simulink model "project"  (R2022b)
settings: Solver=FixedStepDiscrete  StartTime=0.0  StopTime=inf  RelTol=1e-3
undefined symbols (not defined in the file): dfilt, fdesignblkfcn, gcbh
libraries: audiofilters x12, dspsnks4 x6, dsparch4 x6, dspvision x6, dspfdesign x3, simulink x3
settings Model: Creator=KT  LastModifiedBy=KT
settings SolverCC: AlgebraicLoopSolver=TrustRegion  AutoInsertRateTranBlk=on
settings DataIOCC: LimitDataPoints=on  SaveOutput=off  SignalLogging=off  SaveTime=off
settings OptimizationCC: LifeSpan=inf
settings DebuggingCC: AlgebraicLoopMsg=error  SingleTaskRateTransMsg=error  UnconnectedInputMsg=warning  UnconnectedOutputMsg=warning  UnconnectedLineMsg=warning  AllowSymbolicDim=off  SFUnexpectedBacktrackingDiag=warning  SFNoUnconditionalDefaultTransitionDiag=warning  SFExecutionAtInitializationDiag=none  SFMachineParentedDataDiag=warning  ArithmeticOperatorsInVariantConditions=warning
settings ModelReferenceCC: EnableRefExpFcnMdlSchedulingChecks=on
settings SFSimCC: SimUseLocalCustomCode=off  CustomCodeUndefinedFunction=UseInterfaceOnly
settings RTWCC: RTWUseLocalCustomCode=off
settings CodeAppCC: StateflowObjectComments=on
settings GRTTargetCC: TargetLangStandard=C89/C90 (ANSI)
settings ConfigComp: CovMetricSettings=dw  CovSaveCumulativeToWorkspaceVar=on  CovSaveSingleToWorkspaceVar=on  CovExternalEMLEnable=off  CovSFcnEnable=off

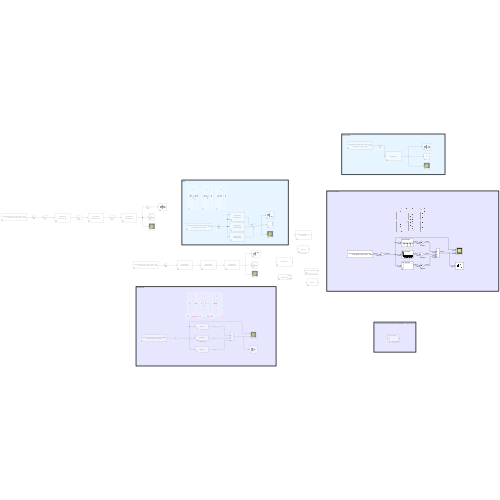
[thumbnail: Simulink's stored preview of the top-level diagram]
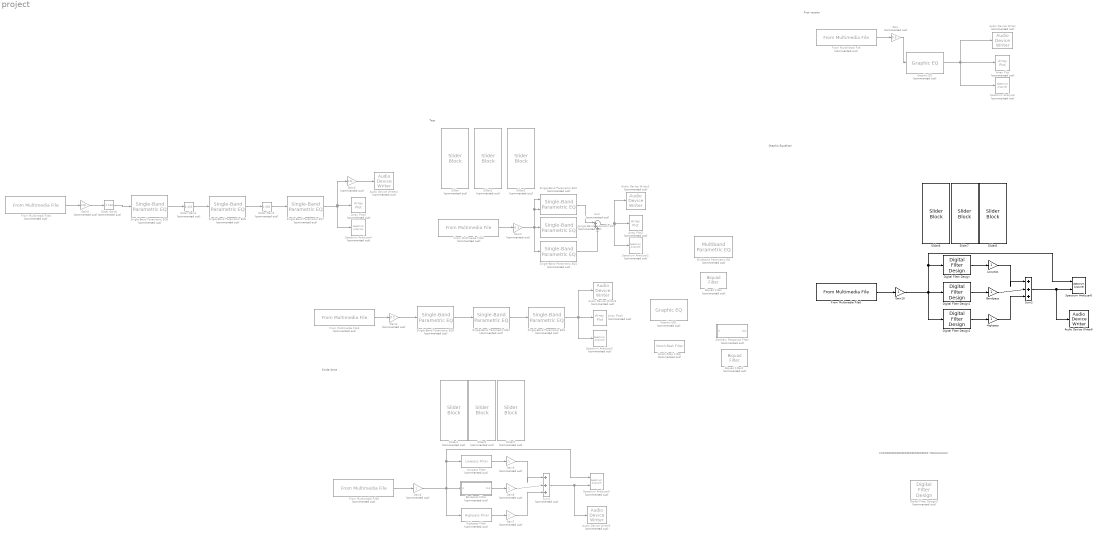
== system project ==
  note: FUCKKKKKKKKKKKKKKKKKKKKKKKKKK YOUUUUUUU!
  note: Kinda done
  note: Graphic Equalizer
  note: First version
  note: Test
  Arbitrary Response Filter : Subsystem  Commented=on  DialogController=fdesignblkfcn  InitFcn=fdesignblkfcn(gcbh, {'InitFcn'});  mask(Arbitrary Magnitude Filter){}
      mask help: Design an arbitrary magnitude filter
      settings: CopyFcn=fdesignblkfcn(gcbh, {'CopyFcn'});
      mask Help: helpview(mapfilelocation('dsp'), 'dsparbitrarymagnitudefilter');
      mask Display: disp('Arbitrary Response');
  Array Plot : ArrayPlot  Commented=on  WindowPosition=[1657.000000,112.000000,800.000000,500.000000,]  ScopeFrameLocation=window  YLimits=[-0.9589,1.0609]  ShowLegend=on
  Array Plot2 : ArrayPlot  Commented=on  WindowPosition=[1657.000000,112.000000,800.000000,500.000000,]  ScopeFrameLocation=window  YLimits=[-0.3932,0.3437]  ShowLegend=on
  Array Plot3 : ArrayPlot  Commented=on  WindowPosition=[1657.000000,112.000000,800.000000,500.000000,]  ScopeFrameLocation=window  YLimits=[-0.0682,0.0646]  ShowLegend=on
  Array Plot4 : ArrayPlot  Commented=on  WindowPosition=[1657.000000,112.000000,800.000000,500.000000,]  ScopeFrameLocation=window  YLimits=[-1.0204,0.9782]  ShowLegend=on
  Audio Device Writer{,2..5} (5 alike) : dspsnks4/Audio Device Writer  Commented=on  Driver=DirectSound  Device=Default  InheritSampleRate=on  SampleRate=44100  BitDepth=16-bit integer  BufferSize=4096  NumBuffers=10  DefaultOutputChannelMapping=on  OutputChannelMapping=1:2  OutputNumUnderrunSamples=off  DriverIdx=1  DeviceWarnFlag=''
  Audio Device Writer6 : dspsnks4/Audio Device Writer  Driver=DirectSound  Device=Default  InheritSampleRate=on  SampleRate=44100  BitDepth=16-bit integer  BufferSize=4096  NumBuffers=10  DefaultOutputChannelMapping=on  OutputChannelMapping=1:2  OutputNumUnderrunSamples=off  DriverIdx=1  DeviceWarnFlag=''
  Bandpass : Gain
  Bandpass Filter : Subsystem  Commented=on  DialogController=fdesignblkfcn  InitFcn=fdesignblkfcn(gcbh, {'InitFcn'});  mask(Bandpass Filter){}
      mask help: Design a bandpass filter
      settings: CopyFcn=fdesignblkfcn(gcbh, {'CopyFcn'});
      mask Help: helpview(mapfilelocation('dsp'), 'dspbandpassfilter');
      mask Display: disp('Bandpass');
  Biquad Filter : dsparch4/Biquad Filter  Commented=on  FilterSource=Dialog parameters  CoeffSource=Specify via dialog  FilterObject=dfilt.df2tsos([1 0.3 0.4],[1 0.1 0.2])  IIRFiltStruct=Direct form II transposed  BiQuadCoeffs=[1 0.3 0.4 1 0.1 0.2]  ScaleValues=1  IC=0  ICnum=0  ICden=0  a0Flag=Warning  optimizeScaleValues=on  ScaleValueMode=Specify via input port (g)  roundingMode=Floor  overflowMode=off  scaleValueFracLength=14  denProdOutputFracLength=30  denAccumFracLength=30  secondMemoryFracLength=15
      settings: LibrarySourceBlock=dsphdlsupportfiltering/Biquad Filter
  Biquad Filter1 : dsparch4/Biquad Filter  Commented=on  FilterSource=Dialog parameters  CoeffSource=Specify via dialog  FilterObject=BQF  IIRFiltStruct=Direct form II transposed  BiQuadCoeffs=[1 0.3 0.4 1 0.1 0.2]  ScaleValues=1  IC=0  ICnum=0  ICden=0  a0Flag=Warning  optimizeScaleValues=on  ScaleValueMode=Specify via input port (g)  InputProcessing=Columns as channels (frame based)  roundingMode=Floor  overflowMode=off  scaleValueFracLength=14  denProdOutputFracLength=30  denAccumFracLength=30  secondMemoryFracLength=15
  Digital Filter Design : dsparch4/Digital Filter Design  mwdsp_browser_bugfix_var=off
  Digital Filter Design1 : dsparch4/Digital Filter Design  mwdsp_browser_bugfix_var=off
  Digital Filter Design2 : dsparch4/Digital Filter Design  mwdsp_browser_bugfix_var=off
  Digital Filter Design3 : dsparch4/Digital Filter Design  Commented=on  mwdsp_browser_bugfix_var=off
  From Multimedia File{,2..5} (5 alike) : dspvision/From Multimedia File  Commented=on  inputFilename=RockGuitar-16-44p1-stereo-72secs.wav  readRange=[1 Inf]  loop=on  numPlays=inf  outputStreams=Audio only  videoDataType=single  audioDataType=double  inheritSampleTime=on  userDefinedSampleTime=1/30  noAudioOutput=off  isIntensityVideo=off  fourcc=RGB  colorVideoFormat=Separate color signals  outputEOF=off  dataOrg=Column-major  audioFrameSize=1024  computeAudioFrameSize=off  outSamplingMode=Sample based
  From Multimedia File6 : dspvision/From Multimedia File  inputFilename=RockGuitar-16-44p1-stereo-72secs.wav  readRange=[1 Inf]  loop=on  numPlays=inf  outputStreams=Audio only  videoDataType=single  audioDataType=double  inheritSampleTime=on  userDefinedSampleTime=1/30  noAudioOutput=off  isIntensityVideo=off  fourcc=RGB  colorVideoFormat=Separate color signals  outputEOF=off  dataOrg=Column-major  audioFrameSize=1024  computeAudioFrameSize=off  outSamplingMode=Sample based
  Gain : Gain  Commented=on  Gain=0.5
  Gain10 : Gain
  Gain2 : Gain  Commented=on  Gain=0.1
  Gain3 : Gain  Commented=on  Gain=0.1
  Gain{4,7..9} (4 alike) : Gain  Commented=on
  Gain5 : Gain  Commented=on  Gain=0.05
  Gain6 : Gain  Commented=on  Gain=0.05
  Graphic EQ : audiofilters/Graphic EQ  Commented=on  EQOrder=2  Bandwidth=1 octave  Structure=Cascade  Gain_25=0  Gain_31_5=-0.800  Gain_40=0  Gain_50=0  Gain_63=8.800  Gain_80=0  Gain_100=0  Gain_125=6.800  Gain_160=0  Gain_200=0  Gain_250=8.800  Gain_315=0  Gain_400=0  Gain_500=11.600  Gain_630=0  Gain_800=0  Gain_1000=5.600  Gain_1250=0  Gain_1600=0  Gain_2000=6.400  Gain_2500=0  Gain_3150=0  Gain_4000=4.400  Gain_5000=0  Gain_6300=0  Gain_8000=0  Gain_10000=0  Gain_12500=0  Gain_16000=-0.800  Gain_20000=0  WorkspaceVariableName=myFilt  OverwriteExportVariable=on  InheritSampleRate=off  SampleRate=44100  SimulateUsing=Code generation
  Graphic EQ1 : audiofilters/Graphic EQ  Commented=on  EQOrder=2  Bandwidth=1 octave  Structure=Cascade  Gain_25=0  Gain_31_5=0  Gain_40=0  Gain_50=0  Gain_63=0  Gain_80=0  Gain_100=0  Gain_125=0  Gain_160=0  Gain_200=0  Gain_250=0  Gain_315=0  Gain_400=0  Gain_500=0  Gain_630=0  Gain_800=0  Gain_1000=0  Gain_1250=0  Gain_1600=0  Gain_2000=0  Gain_2500=0  Gain_3150=0  Gain_4000=0  Gain_5000=0  Gain_6300=0  Gain_8000=0  Gain_10000=0  Gain_12500=0  Gain_16000=0  Gain_20000=0  WorkspaceVariableName=myFilt  OverwriteExportVariable=on  InheritSampleRate=off  SampleRate=44100  SimulateUsing=Code generation
  Highpass : Gain
  Highpass Filter : dspfdesign/Highpass Filter  Commented=on  FilterType=FIR  DesignForMinimumOrder=on  FilterOrder=100  StopbandFrequency=3000  PassbandFrequency=4000  StopbandAttenuation=40  PassbandRipple=0.5  InheritSampleRate=off  SampleRate=44100  SimulateUsing=Interpreted execution  roundingMode=Floor  coeffsDataTypeStr=fixdt(1,16)
  Lowpass : Gain
  Lowpass Filter : dspfdesign/Lowpass Filter  Commented=on  FilterType=FIR  DesignForMinimumOrder=on  FilterOrder=100  PassbandFrequency=125  StopbandFrequency=250  PassbandRipple=0.5  StopbandAttenuation=40  InheritSampleRate=off  SampleRate=44100  SimulateUsing=Interpreted execution  roundingMode=Floor  coeffsDataTypeStr=fixdt(1,16)
  Multiband Parametric EQ : audiofilters/Multiband Parametric EQ  Commented=on  EQOrder=2  NumEQBands=3  FrequenciesPort=off  Frequencies=[100 181 325]  PeakGainsPort=off  PeakGains=[0 0 0]  QualityFactorsPort=off  QualityFactors=[1.6 1.6 1.6]  InheritSampleRate=off  SampleRate=44100  WorkspaceVariableName=myFilt  OverwriteExportVariable=on  HasLowShelfFilter=off  LowShelfCutoffPort=off  LowShelfCutoff=200  LowShelfSlopePort=off  LowShelfSlope=1.5  LowShelfGainPort=off  LowShelfGain=0  HasHighShelfFilter=off  HighShelfCutoffPort=off  HighShelfCutoff=15e3  HighShelfSlopePort=off  HighShelfSlope=1.5  HighShelfGainPort=off  HighShelfGain=0  HasLowpassFilter=off  LowpassCutoffPort=off  LowpassCutoff=18e3  LowpassSlopePort=off  LowpassSlope=12  HasHighpassFilter=off  HighpassCutoffPort=off  HighpassCutoff=20  HighpassSlopePort=off  HighpassSlope=30  Oversample=off  SimulateUsing=Code generation
  Notch-Peak Filter : dspfdesign/Notch-Peak Filter  Commented=on  Specification=Bandwidth and center frequency  BandwidthPort=off  Bandwidth=2205  QualityFactorPort=off  QualityFactor=5  CenterFrequencyPort=off  CenterFrequency=11025  BandwidthCoefficientPort=off  BandwidthCoefficient=0.72654  CenterFrequencyCoefficientPort=off  CenterFrequencyCoefficient=0  Output=Notch and Peak  InheritSampleRate=off  SampleRate=44100  SimulateUsing=Code generation
  Single-Band Parametric EQ : audiofilters/Single-Band Parametric EQ  Commented=on  FilterOrder=2  Specification=Bandwidth and center frequency  CenterFrequencyPort=off  CenterFrequency=600.0  BandwidthPort=off  Bandwidth=1200.0  QualityFactorPort=off  QualityFactor=5  PeakGaindBPort=off  PeakGaindB=0  InheritSampleRate=off  SampleRate=44100  SimulateUsing=Code generation
  Single-Band Parametric EQ1 : audiofilters/Single-Band Parametric EQ  Commented=on  FilterOrder=2  Specification=Bandwidth and center frequency  CenterFrequencyPort=off  CenterFrequency=600.0  BandwidthPort=off  Bandwidth=1200.0  QualityFactorPort=off  QualityFactor=5  PeakGaindBPort=off  PeakGaindB=0  InheritSampleRate=off  SampleRate=44100  SimulateUsing=Code generation
  Single-Band Parametric EQ2 : audiofilters/Single-Band Parametric EQ  Commented=on  FilterOrder=2  Specification=Bandwidth and center frequency  CenterFrequencyPort=off  CenterFrequency=600.0  BandwidthPort=off  Bandwidth=1200.0  QualityFactorPort=off  QualityFactor=5  PeakGaindBPort=on  PeakGaindB=0  InheritSampleRate=off  SampleRate=44100  SimulateUsing=Code generation
  Single-Band Parametric EQ3 : audiofilters/Single-Band Parametric EQ  Commented=on  FilterOrder=2  Specification=Quality factor and center frequency  CenterFrequencyPort=off  CenterFrequency=1000  BandwidthPort=off  Bandwidth=0.3  QualityFactorPort=off  QualityFactor=0.498  PeakGaindBPort=off  PeakGaindB=0.0  InheritSampleRate=off  SampleRate=44100  SimulateUsing=Code generation
  Single-Band Parametric EQ4 : audiofilters/Single-Band Parametric EQ  Commented=on  FilterOrder=2  Specification=Quality factor and center frequency  CenterFrequencyPort=off  CenterFrequency=4000.0  BandwidthPort=off  Bandwidth=800.0  QualityFactorPort=off  QualityFactor=0.7  PeakGaindBPort=off  PeakGaindB=0.0  InheritSampleRate=off  SampleRate=44100  SimulateUsing=Code generation
  Single-Band Parametric EQ5 : audiofilters/Single-Band Parametric EQ  Commented=on  FilterOrder=2  Specification=Quality factor and center frequency  CenterFrequencyPort=off  CenterFrequency=250  BandwidthPort=off  Bandwidth=3800.0  QualityFactorPort=off  QualityFactor=0.7  PeakGaindBPort=off  PeakGaindB=0.0  InheritSampleRate=off  SampleRate=44100  SimulateUsing=Code generation
  Single-Band Parametric EQ6 : audiofilters/Single-Band Parametric EQ  Commented=on  FilterOrder=2  Specification=Quality factor and center frequency  CenterFrequencyPort=off  CenterFrequency=1000  BandwidthPort=off  Bandwidth=0.3  QualityFactorPort=off  QualityFactor=0.498  PeakGaindBPort=off  PeakGaindB=0  InheritSampleRate=off  SampleRate=44100  SimulateUsing=Code generation
  Single-Band Parametric EQ7 : audiofilters/Single-Band Parametric EQ  Commented=on  FilterOrder=2  Specification=Quality factor and center frequency  CenterFrequencyPort=off  CenterFrequency=4000.0  BandwidthPort=off  Bandwidth=800.0  QualityFactorPort=off  QualityFactor=0.7  PeakGaindBPort=off  PeakGaindB=0  InheritSampleRate=off  SampleRate=44100  SimulateUsing=Code generation
  Single-Band Parametric EQ8 : audiofilters/Single-Band Parametric EQ  Commented=on  FilterOrder=2  Specification=Quality factor and center frequency  CenterFrequencyPort=off  CenterFrequency=250  BandwidthPort=off  Bandwidth=3800.0  QualityFactorPort=off  QualityFactor=0.7  PeakGaindBPort=off  PeakGaindB=0  InheritSampleRate=off  SampleRate=44100  SimulateUsing=Code generation
  Slider : SliderBlock  Commented=on
  Slider Gain4 : simulink/Math Operations/Slider Gain  Commented=on  gain=8.400  low=-12  high=12
  Slider Gain5 : simulink/Math Operations/Slider Gain  Commented=on  gain=1.680  low=-12  high=12
  Slider Gain6 : simulink/Math Operations/Slider Gain  Commented=on  gain=2.160  low=-12  high=12
  Slider1 : SliderBlock  Commented=on
  Slider2 : SliderBlock  Commented=on
  Slider3 : SliderBlock  Commented=on  ScaleMin=-12  ScaleMax=12
  Slider4 : SliderBlock  Commented=on  ScaleMin=-12  ScaleMax=12
  Slider5 : SliderBlock  Commented=on  ScaleMin=-12  ScaleMax=12
  Slider6 : SliderBlock  ScaleMin=-12  ScaleMax=12
  Slider7 : SliderBlock  ScaleMin=-12  ScaleMax=12
  Slider8 : SliderBlock  ScaleMin=-12  ScaleMax=12
  Spectrum Analyzer{,2..4} (4 alike) : SpectrumAnalyzer  Commented=on
  Spectrum Analyzer5 : SpectrumAnalyzer  Commented=on  NumInputPorts=2
  Spectrum Analyzer6 : SpectrumAnalyzer  NumInputPorts=2
  Sum : Sum  Commented=on  Inputs=|+++
  Sum1 : Sum  Commented=on  Inputs=|+++
  Sum2 : Sum  Inputs=|+++
  wires:
  From Multimedia File/1 -> Gain/1
  Graphic EQ/1 -> Audio Device Writer/1, Spectrum Analyzer/1, Array Plot/1
  Gain/1 -> Graphic EQ/1
  Gain2/1 -> Single-Band Parametric EQ1/1, Single-Band Parametric EQ2/2, Single-Band Parametric EQ2/1, Single-Band Parametric EQ/1
  From Multimedia File2/1 -> Gain2/1
  Single-Band Parametric EQ2/1 -> Sum/1
  Single-Band Parametric EQ/1 -> Sum/2
  Single-Band Parametric EQ1/1 -> Sum/3
  Sum/1 -> Audio Device Writer2/1, Array Plot2/1, Spectrum Analyzer2/1
  Single-Band Parametric EQ4/1 -> Audio Device Writer3/1, Array Plot3/1, Spectrum Analyzer3/1
  From Multimedia File3/1 -> Gain3/1
  Slider Gain5/1 -> Single-Band Parametric EQ7/1
  Single-Band Parametric EQ6/1 -> Slider Gain5/1
  Slider Gain4/1 -> Single-Band Parametric EQ6/1
  Single-Band Parametric EQ8/1 -> Slider Gain4/1
  Slider Gain6/1 -> Single-Band Parametric EQ8/1
  Gain5/1 -> Slider Gain6/1
  Gain6/1 -> Audio Device Writer4/1
  From Multimedia File4/1 -> Gain5/1
  Single-Band Parametric EQ7/1 -> Spectrum Analyzer4/1, Gain6/1, Array Plot4/1
  Single-Band Parametric EQ3/1 -> Single-Band Parametric EQ4/1
  Single-Band Parametric EQ5/1 -> Single-Band Parametric EQ3/1
  Gain3/1 -> Single-Band Parametric EQ5/1
  From Multimedia File5/1 -> Gain4/1
  Gain4/1 -> Lowpass Filter/1, Spectrum Analyzer5/1, Bandpass Filter/1(In), Highpass Filter/1
  Highpass Filter/1 -> Gain7/1
  Gain8/1 -> Sum1/2
  Gain9/1 -> Sum1/1
  Gain7/1 -> Sum1/3
  Sum1/1 -> Audio Device Writer5/1, Spectrum Analyzer5/2
  Bandpass Filter/1(Out) -> Gain8/1
  Lowpass Filter/1 -> Gain9/1
  Digital Filter Design/1 -> Lowpass/1
  Digital Filter Design1/1 -> Bandpass/1
  Sum2/1 -> Spectrum Analyzer6/2, Audio Device Writer6/1
  Highpass/1 -> Sum2/3
  Lowpass/1 -> Sum2/1
  Bandpass/1 -> Sum2/2
  Digital Filter Design2/1 -> Highpass/1
  Gain10/1 -> Digital Filter Design2/1, Digital Filter Design1/1, Digital Filter Design/1, Spectrum Analyzer6/1
  From Multimedia File6/1 -> Gain10/1

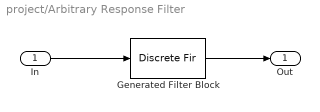
== system project/Arbitrary Response Filter ==
  In : Inport
  Generated Filter Block : DiscreteFir  Tag=BlockMethodSubSystem  Coefficients=[-6.05289744107923022e-17 -0.0303024499678175019 5.57990532024364168e-18 -0.0423165804135848464 1.96303886531922274e-17 -0.1094403863154082 6.51513653930646848e-17 0.286668225801437471 -9.07686891479065023e-17 0.0937838026666719948 0.5 0.0937838026666717173 1.48637050553399557e-16 0.286668225801437471 -1.18208343547727341e-16 -0.109440386315408089 3.11708124589582525e-17 -0.0423165804135848256 -8.11286903003504086e-17 -0.0303024499678174464 1.20107567778704496e-16]  InputProcessing=Columns as channels (frame based)
  Out : Outport  VectorParamsAs1DForOutWhenUnconnected=off
  wires:
  Generated Filter Block/1 -> Out/1
  In/1 -> Generated Filter Block/1

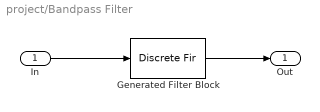
== system project/Bandpass Filter ==
  In : Inport
  Generated Filter Block : DiscreteFir  Tag=BlockMethodSubSystem  Coefficients=[-0.191129939643672114 -0.04182100165159746 -0.0324519768568180614 -0.0150380352860095112 0.00653823963646311609 0.026896052555044115 0.040494078194709085 0.0431305328870113802 0.0331784454415686922 0.0121749667915446395 -0.0152466702751226906 -0.0424978780273151599 -0.0623837933939399847 -0.0692732368320401609 -0.0604779206578360193 -0.0371922014776995824 -0.00458597343800470035 0.0294305519946282748 0.0561441356804084149 0.0682742687712988849 0.0618561048814014816 0.0376537397670379317 0.00090093281973986064 -0.0396474587773330972 -0.0739486415173737782 -0.0929641748347522223 -0.0911678669850860823 -0.0681881203261401891 -0.0293003206038559144 0.016326057004679824 0.0580541067989199314 0.0844735689750536756 0.089260026256607311 0.07032904329684736 0.0318391430830373412 -0.0173067385941670718 -0.0654033193039453703 -0.100910712901346039 -0.115232846295472161 -0.104765858762353239 -0.0718237988802253452 -0.0236480524314124606 0.0289621370824939689 0.0751260484389913857 0.106161109927425626 0.117698851870551346 0.110850256361664207 0.0913797774695053466 0.0678925100779304569 0.0492671718662415423 0.0422524483589877958 0.0492671718662415423 0.0678925100779304569 0.0913797774695053466 0.110850256361664207 0.117698851870551346 0.106161109927425626 0.0751260484389913857 0.0289621370824939689 -0.0236480524314124606 -0.0718237988802253452 -0.104765858762353239 -0.115232846295472161 -0.100910712901346039 -0.0654033193039453703 -0.0173067385941670718 0.0318391430830373412 0.07032904329684736 0.089260026256607311 0.0844735689750536756 0.0580541067989199314 0.016326057004679824 -0.0293003206038559144 -0.0681881203261401891 -0.0911678669850860823 -0.0929641748347522223 -0.0739486415173737782 -0.0396474587773330972 0.00090093281973986064 0.0376537397670379317 0.0618561048814014816 0.0682742687712988849 0.0561441356804084149 0.0294305519946282748 -0.00458597343800470035 -0.0371922014776995824 -0.0604779206578360193 -0.0692732368320401609 -0.0623837933939399847 -0.0424978780273151599 -0.0152466702751226906 0.0121749667915446395 0.0331784454415686922 0.0431305328870113802 0.040494078194709085 0.026896052555044115 0.00653823963646311609 -0.0150380352860095112 -0.0324519768568180614 -0.04182100165159746 -0.191129939643672114]  InputProcessing=Columns as channels (frame based)
  Out : Outport  VectorParamsAs1DForOutWhenUnconnected=off
  wires:
  In/1 -> Generated Filter Block/1
  Generated Filter Block/1 -> Out/1
